simulink model "kers_discharge_versione_2019a"  (R2019b)
settings: Solver=FixedStepAuto  StartTime=0.0  StopTime=50  FixedStep=0.0001  MinStep=0.00001  RelTol=1e-3
values from neighbouring files (symbols this model uses):
  d = 0.49    [Data.m]
  Jeq_v = 120    [Data.m]
  Jf = 0.026    [Data.m]
  tau_max = 2.5    [Data.m]
  tau_min = 0.4    [Data.m]
  tau_trasm = 62.8    [Data.m]
  Tmax = 240    [Data.m]
  wf_max = 60000/9.55    (= 6282.72251309)    [Data.m]
undefined symbols (not defined in the file or in its folder): Rw, tau1, tau2, tau3, tau4, tau5, tau6, tau7, tauf, V1max, V2max, V3max, V4max, V5max, V6max
libraries: simulink x2
settings Model: Creator=andre  LastModifiedBy=Luca
settings SolverCC: ZeroCrossAlgorithm=Adaptive
settings DebuggingCC: IgnoredZcDiagnostic=none
settings SFSimCC: CustomCodeUndefinedFunction=UseInterfaceOnly

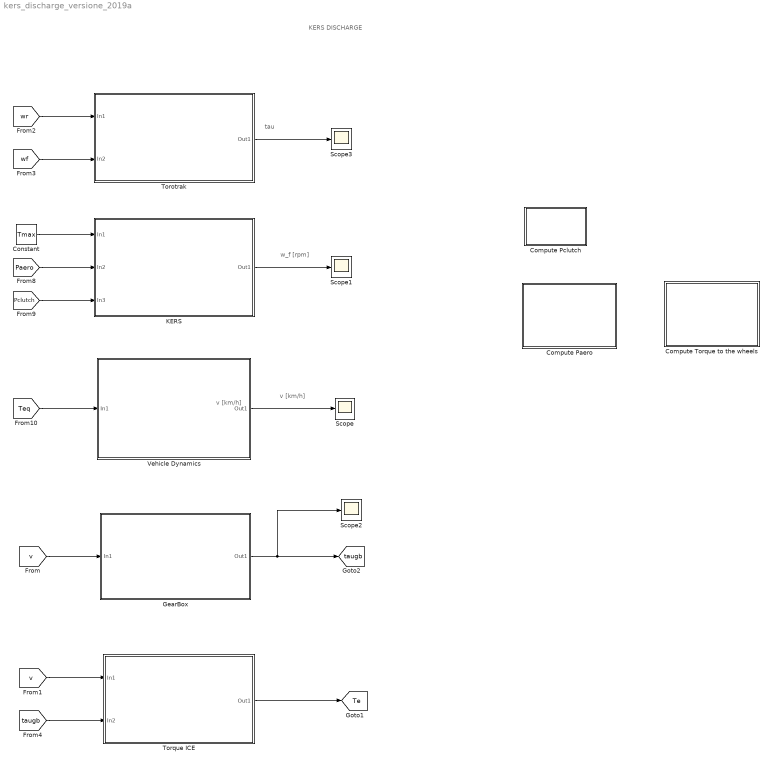
== system kers_discharge_versione_2019a ==
  note: KERS DISCHARGE
  note: v [km/h]
  note: w_f [rpm]
  note: v [km/h]
  note: tau
  Compute Paero : Subsystem
  Compute Pclutch : Subsystem
  Compute Torque to the wheels : Subsystem
  Constant : Constant  Value=Tmax  SampleTime=-1
  GearBox : Subsystem
      mask Display: image("GearBox.jpg")
  KERS : Subsystem
      mask Display: image('KERS.jpg'); % Use "Edit Image" on toolstrip to change.
  Scope{,1..3} (4 alike) : Scope
  Torotrak : Subsystem
      mask Display: image('Torotrak.jpg'); % Use "Edit Image" on toolstrip to change.
  Torque ICE : Subsystem
      mask Display: image("ICE.jpg")
  Vehicle Dynamics : Subsystem
      mask Display: image('Ferrari.jpg'); % Use "Edit Image" on toolstrip to change.
  tag scope: Te=global, taugb=global
  wires:
  [wr] -> Torotrak/1(In1)
  [wf] -> Torotrak/2(In2)
  Torotrak/1(Out1) -> Scope3/1
  [Teq] -> Vehicle Dynamics/1(In1)
  Vehicle Dynamics/1(Out1) -> Scope/1
  [Paero] -> KERS/2(In2)
  [Pclutch] -> KERS/3(In3)
  KERS/1(Out1) -> Scope1/1
  [v] -> GearBox/1(In1)
  GearBox/1(Out1) -> [taugb], Scope2/1
  [v] -> Torque ICE/1(In1)
  [taugb] -> Torque ICE/2(In2)
  Torque ICE/1(Out1) -> [Te]
  Constant/1 -> KERS/1(In1)

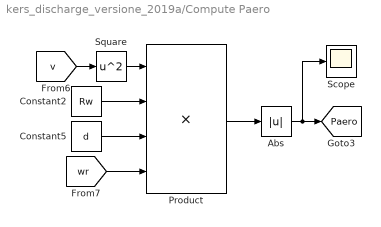
== system kers_discharge_versione_2019a/Compute Paero ==
  Abs : Abs
  Constant2 : Constant  Value=Rw
  Constant5 : Constant  Value=d
  Product : Product  Inputs=4
  Scope : Scope
  Square : Math  Operator=square  SignedPower=on  OutputSignalType=real  SaturateOnIntegerOverflow=on
  tag scope: Paero=global
  wires:
  Square/1 -> Product/1
  Constant5/1 -> Product/3
  [wr] -> Product/4
  [v] -> Square/1
  Constant2/1 -> Product/2
  Product/1 -> Abs/1
  Abs/1 -> Scope/1, [Paero]

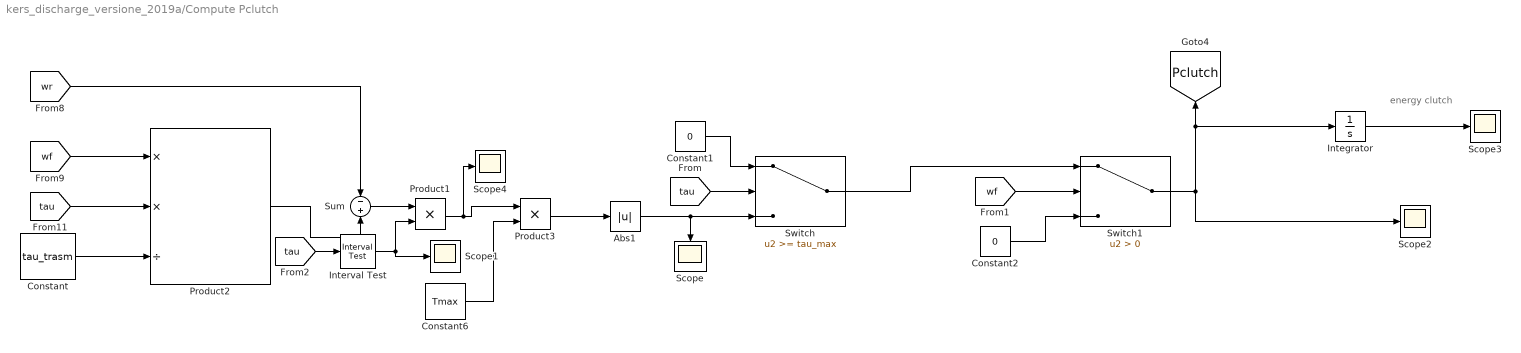
== system kers_discharge_versione_2019a/Compute Pclutch ==
  note: energy clutch
  Abs1 : Abs  ZeroCross=off
  Constant : Constant  Value=tau_trasm
  Constant1 : Constant  Value=0
  Constant2 : Constant  Value=0
  Constant6 : Constant  Value=Tmax
  Integrator : Integrator
  Interval Test : simulink/Logic and Bit Operations/Interval Test  IntervalClosedRight=on  uplimit=tau_max-0.1  IntervalClosedLeft=on  lowlimit=0.4  OutDataTypeStr=boolean
  Product1 : Product
  Product2 : Product  Inputs=**/
  Product3 : Product
  Scope{,1..4} (5 alike) : Scope
  Sum : Sum  Inputs=-+
  Switch : Switch  Threshold=tau_max
  Switch1 : Switch  Criteria=u2 > Threshold
  tag scope: Pclutch=global
  wires:
  Product2/1 -> Sum/2
  [wf] -> Product2/1
  Constant6/1 -> Product3/2
  [wr] -> Sum/1
  Constant/1 -> Product2/3
  [tau] -> Product2/2
  Product3/1 -> Abs1/1
  [tau] -> Switch/2
  [wf] -> Switch1/2
  Integrator/1 -> Scope3/1
  Switch1/1 -> Scope2/1, Integrator/1, [Pclutch]
  Constant1/1 -> Switch/1
  Abs1/1 -> Scope/1, Switch/3
  Switch/1 -> Switch1/1
  Constant2/1 -> Switch1/3
  [tau] -> Interval Test/1
  Sum/1 -> Product1/1
  Interval Test/1 -> Product1/2, Scope1/1
  Product1/1 -> Scope4/1, Product3/1

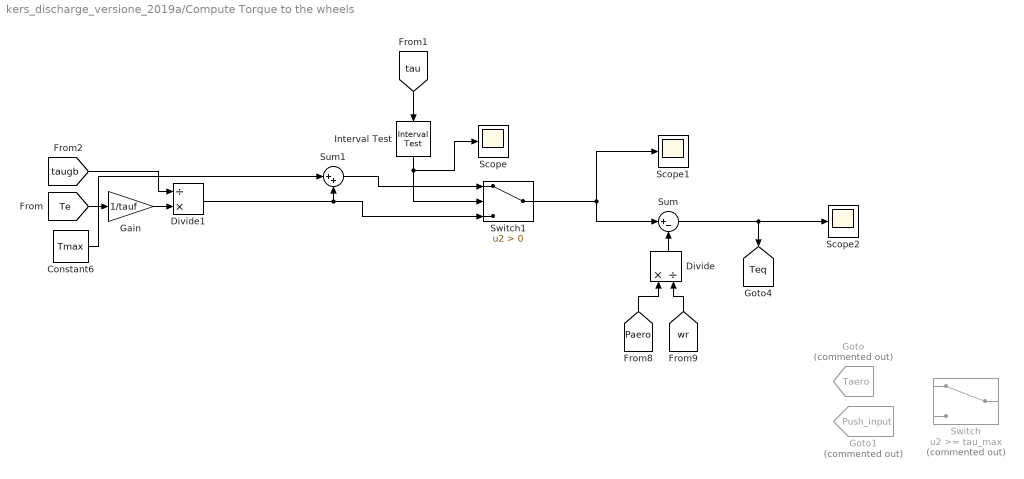
== system kers_discharge_versione_2019a/Compute Torque to the wheels ==
  Constant6 : Constant  Value=Tmax
  Divide : Product  Inputs=*/
  Divide1 : Product  Inputs=/*
  Gain : Gain  Gain=1/tauf
  Goto : Goto  Commented=on  GotoTag=Taero  TagVisibility=global
  Goto1 : Goto  Commented=on  GotoTag=Push_input  TagVisibility=global
  Interval Test : simulink/Logic and Bit Operations/Interval Test  IntervalClosedRight=on  uplimit=tau_max-0.00001  IntervalClosedLeft=on  lowlimit=0.4  OutDataTypeStr=boolean
  Scope : Scope
  Scope1 : Scope
  Scope2 : Scope
  Sum : Sum  Inputs=|+-
  Sum1 : Sum  Inputs=|++
  Switch : Switch  Commented=on  Threshold=tau_max
  Switch1 : Switch  Criteria=u2 > Threshold
  tag scope: Teq=global
  wires:
  Sum/1 -> Scope2/1, [Teq]
  [Paero] -> Divide/1
  [wr] -> Divide/2
  Divide/1 -> Sum/2
  [Te] -> Gain/1
  Gain/1 -> Divide1/2
  [taugb] -> Divide1/1
  [tau] -> Interval Test/1
  Interval Test/1 -> Scope/1, Switch1/2
  Divide1/1 -> Sum1/2, Switch1/3
  Switch1/1 -> Sum/1, Scope1/1
  Constant6/1 -> Sum1/1
  Sum1/1 -> Switch1/1

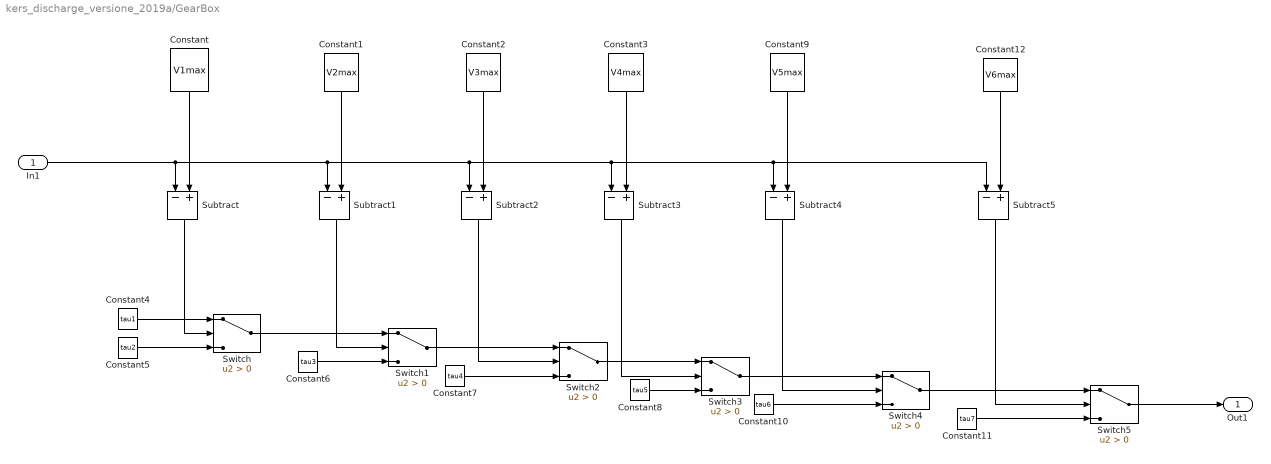
== system kers_discharge_versione_2019a/GearBox ==
  In1 : Inport
  Constant : Constant  Value=V1max
  Constant1 : Constant  Value=V2max
  Constant10 : Constant  Value=tau6
  Constant11 : Constant  Value=tau7
  Constant12 : Constant  Value=V6max
  Constant2 : Constant  Value=V3max
  Constant3 : Constant  Value=V4max
  Constant4 : Constant  Value=tau1
  Constant5 : Constant  Value=tau2
  Constant6 : Constant  Value=tau3
  Constant7 : Constant  Value=tau4
  Constant8 : Constant  Value=tau5
  Constant9 : Constant  Value=V5max
  Subtract{,1..5} (6 alike) : Sum  Inputs=-+
  Switch{,1..5} (6 alike) : Switch  Criteria=u2 > Threshold
  Out1 : Outport  VectorParamsAs1DForOutWhenUnconnected=off
  wires:
  Constant/1 -> Subtract/2
  In1/1 -> Subtract/1, Subtract1/1, Subtract2/1, Subtract3/1, Subtract4/1, Subtract5/1
  Constant1/1 -> Subtract1/2
  Constant2/1 -> Subtract2/2
  Constant3/1 -> Subtract3/2
  Subtract/1 -> Switch/2
  Constant4/1 -> Switch/1
  Constant5/1 -> Switch/3
  Subtract1/1 -> Switch1/2
  Switch/1 -> Switch1/1
  Constant6/1 -> Switch1/3
  Switch1/1 -> Switch2/1
  Subtract2/1 -> Switch2/2
  Constant7/1 -> Switch2/3
  Switch2/1 -> Switch3/1
  Subtract3/1 -> Switch3/2
  Constant8/1 -> Switch3/3
  Constant9/1 -> Subtract4/2
  Subtract4/1 -> Switch4/2
  Switch3/1 -> Switch4/1
  Constant10/1 -> Switch4/3
  Constant11/1 -> Switch5/3
  Constant12/1 -> Subtract5/2
  Subtract5/1 -> Switch5/2
  Switch4/1 -> Switch5/1
  Switch5/1 -> Out1/1

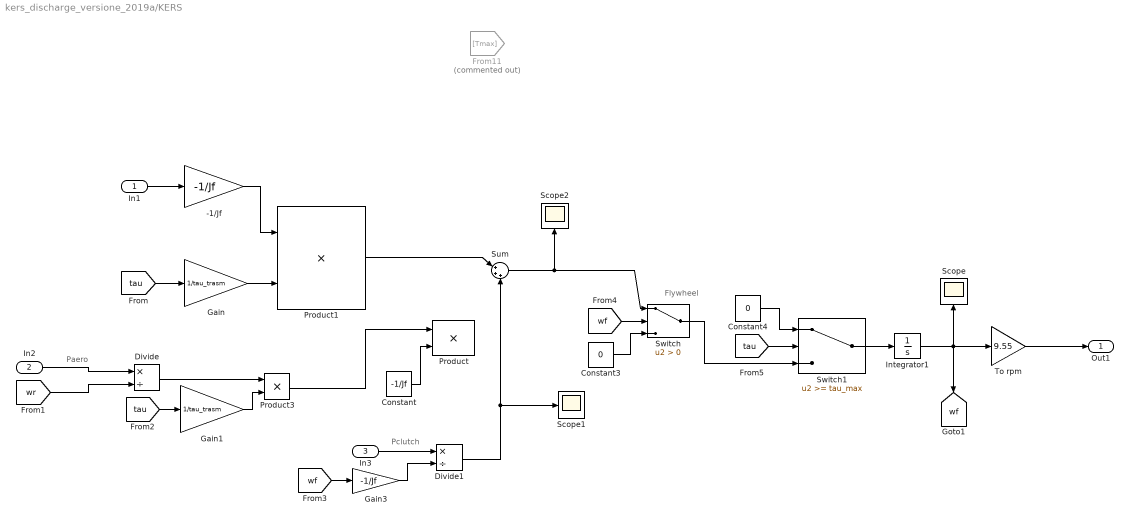
== system kers_discharge_versione_2019a/KERS ==
  note: Pclutch
  note: Paero
  note: Flywheel
  In1 : Inport
  In2 : Inport  Port=2
  In3 : Inport  Port=3
  -1/Jf : Gain  Gain=-1/Jf
  Constant : Constant  Value=-1/Jf
  Constant3 : Constant  Value=0
  Constant4 : Constant  Value=0
  Divide : Product  Inputs=*/
  Divide1 : Product  Inputs=*/
  From11 : From  Commented=on  GotoTag=Tmax  TagVisibility=global
  Gain : Gain  Gain=1/tau_trasm
  Gain1 : Gain  Gain=1/tau_trasm
  Gain3 : Gain  Gain=-1/Jf
  Integrator1 : Integrator  InitialCondition=wf_max  ContinuousStateAttributes="\"omega_f\""
  Product : Product  Inputs=**
  Product1 : Product  Inputs=**
  Product3 : Product
  Scope : Scope
  Scope1 : Scope
  Scope2 : Scope
  Sum : Sum  Inputs=|+++
  Switch : Switch  Criteria=u2 > Threshold
  Switch1 : Switch  Threshold=tau_max
  To rpm : Gain  Gain=9.55
  Out1 : Outport
  tag scope: wf=global
  wires:
  Switch1/1 -> Integrator1/1
  -1/Jf/1 -> Product1/1
  Integrator1/1 -> Scope/1, To rpm/1, [wf]
  [wf] -> Switch/2
  [tau] -> Switch1/2
  Product1/1 -> Sum/1
  To rpm/1 -> Out1/1
  In1/1 -> -1/Jf/1
  Gain/1 -> Product1/2
  [tau] -> Gain/1
  In2/1 -> Divide/1
  [wr] -> Divide/2
  Divide/1 -> Product3/1
  [tau] -> Gain1/1
  Gain1/1 -> Product3/2
  Product3/1 -> Product/1
  Constant/1 -> Product/2
  In3/1 -> Divide1/1
  [wf] -> Gain3/1
  Gain3/1 -> Divide1/2
  Divide1/1 -> Sum/3, Scope1/1
  Constant3/1 -> Switch/3
  Constant4/1 -> Switch1/1
  Switch/1 -> Switch1/3
  Sum/1 -> Scope2/1, Switch/1

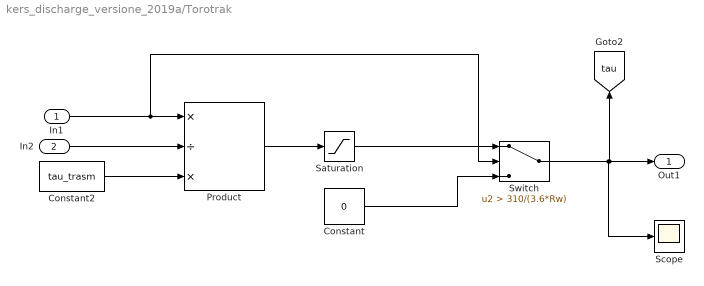
== system kers_discharge_versione_2019a/Torotrak ==
  In1 : Inport
  In2 : Inport  Port=2
  Constant : Constant  Value=0
  Constant2 : Constant  Value=tau_trasm
  Product : Product  Inputs=*/*
  Saturation : Saturate  UpperLimit=tau_max  LowerLimit=tau_min  ZeroCross=off  RndMeth=Nearest
  Scope : Scope
  Switch : Switch  Criteria=u2 > Threshold  Threshold=310/(3.6*Rw)  ZeroCross=off
  Out1 : Outport
  tag scope: tau=global
  wires:
  Constant2/1 -> Product/3
  In1/1 -> Product/1, Switch/2
  In2/1 -> Product/2
  Product/1 -> Saturation/1
  Constant/1 -> Switch/3
  Switch/1 -> Scope/1, [tau], Out1/1
  Saturation/1 -> Switch/1

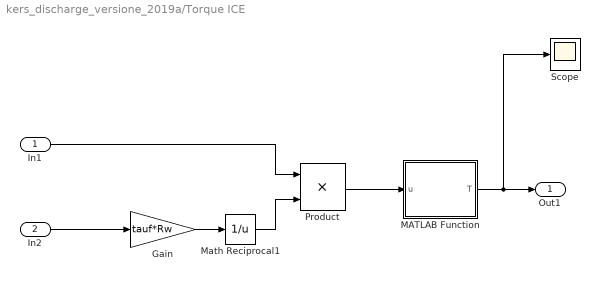
== system kers_discharge_versione_2019a/Torque ICE ==
  In1 : Inport
  In2 : Inport  Port=2
  Gain : Gain  Gain=tauf*Rw
  MATLAB Function : MATLAB Function  TreatAsAtomicUnit=on
  Math Reciprocal1 : Math  Operator=reciprocal  SignedPower=on  SaturateOnIntegerOverflow=on
  Product : Product
  Scope : Scope
  Out1 : Outport  VectorParamsAs1DForOutWhenUnconnected=off
  wires:
  In2/1 -> Gain/1
  Gain/1 -> Math Reciprocal1/1
  Math Reciprocal1/1 -> Product/2
  In1/1 -> Product/1
  MATLAB Function/1(T) -> Scope/1, Out1/1
  Product/1 -> MATLAB Function/1(u)

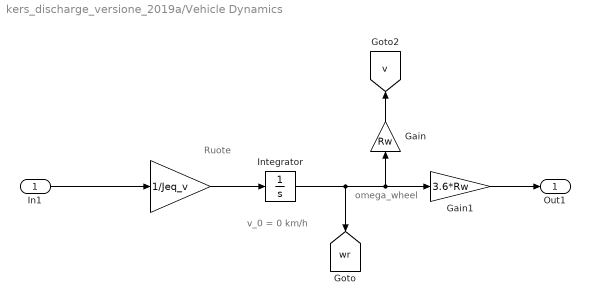
== system kers_discharge_versione_2019a/Vehicle Dynamics ==
  note: omega_wheel
  note: v_0 = 0 km/h
  note: Ruote
  In1 : Inport
  " " : Gain  Gain=1/Jeq_v
  Gain : Gain  Gain=Rw
  Gain1 : Gain  Gain=3.6*Rw
  Integrator : Integrator  InitialCondition=0.000001  ContinuousStateAttributes="\"omega_w\""
  Out1 : Outport
  tag scope: v=global, wr=global
  wires:
  Integrator/1 -> Gain/1, Gain1/1, [wr]
  In1/1 -> " "/1
  Gain/1 -> [v]
  " "/1 -> Integrator/1
  Gain1/1 -> Out1/1

== matlab function kers_discharge_versione_2019a/Torque ICE/MATLAB Function ==
  data: u input; T output
function T = TorqueICE(u)

a0 = 88.48;
a1 = 1.41;
a2 = -8.36e-4;

T = a0+a1*u+a2*(u^2);
